simulink model "eBooster_48v_Gen2_r2009a"  (Simulink 7.6)
settings: Solver=FixedStepDiscrete  StartTime=0.0  StopTime=0.2  FixedStep=T_sim  RelTol=1e-3
InitFcn:
  | init_simulation
values from neighbouring files (symbols this model uses):
  C_Load = 0    [init_MIL.m]    (also in init_simulation.m)
  curr_adc_gain = 0.6247    [init_MIL.m]    (also in init_simulation.m)
  en_avr = 0    [init_MIL.m]    (also in init_simulation.m)
  FOC_CURR_GAIN_SCU10 = 640    [init_MIL.m]    (also in init_simulation.m)
  FOC_CURR_NULLIFICATION = 511    [init_MIL.m]    (also in init_simulation.m)
  I_max = 106    [init_MIL.m]    (also in init_simulation.m = 100; plot_current_limits.m = 160)
  Id_ref_min = -1*160*0.8    (= -128)    [init_MIL.m]    (also in init_simulation.m)
  J_motor = (3.2220 + 11.438)*1e-6    (= 1.466e-05)    [init_MIL.m]    (also in init_simulation.m)
  Kpi = 0.3    [init_MIL.m]    (also in init_simulation.m)
  Kpi_n = 0.0015    [init_MIL.m]    (also in init_simulation.m)
  load_motor_spd_ramp = (load_motor_target_spd - load_motor_start_spd)/spd_ramp_time    (= 62831.8530718)    [init_MIL.m]    (also in init_simulation.m)
  load_motor_start_spd = 40000*2*pi/60    (= 4188.79020479)    [init_MIL.m]    (also in init_simulation.m)
  load_motor_target_spd = 70000*2*pi/60    (= 7330.38285838)    [init_MIL.m]    (also in init_simulation.m)
  Ls = 17.05e-6/3    (= 5.68333333333e-06)    [init_MIL.m]    (also in init_simulation.m; plot_current_limits.m)
  N_avr = 1    [init_MIL.m]    (also in init_simulation.m)
  Nset_const = 50000    [init_MIL.m]    (also in init_simulation.m)
  ONEDIVSQRT3_SCU16 = 37837    [init_MIL.m]    (also in init_simulation.m)
  Pp = 1    [init_MIL.m]    (also in init_simulation.m; plot_current_limits.m)
  psi_p = 5.3e-3/sqrt(3)*0.95    [init_MIL.m]    (also in init_simulation.m)
  Rs = 10e-3*(1+0.0039*(120-20))/3    (= 0.00463333333333)    [init_MIL.m]    (also in init_simulation.m; plot_current_limits.m)
  Sel_Bench_Mode = 1    [init_MIL.m]    (also in init_simulation.m)
  Sel_Bench_Spd = 0    [init_MIL.m]    (also in init_simulation.m)
  Sel_id_ref = 2    [init_MIL.m]    (also in init_simulation.m)
  Sel_Load = 1    [init_MIL.m]    (also in init_simulation.m)
  sel_udq = 0    [init_simulation.m]
  Set_Speed_rpm = 50000    [init_MIL.m]    (also in init_simulation.m)
  T_ctrl = T_pwm    (= 3.57002606119e-05)    [init_MIL.m]    (also in init_simulation.m)
  T_LUT_T = [0.1864, 0.1969, 0.2092, 0.2230, 0.2381, 0.2541, 0.2709, 0.2880, 0.3054, 0.3226, 0.3395, 0.3557, 0.3710, 0.3851, 0.3978, 0.4088, 0.4178 ... (first row only)    [init_MIL.m]    (also in init_simulation.m)
  T_sim = T_pwm/100    (= 3.57002606119e-07)    [init_MIL.m]    (also in init_simulation.m)
  Tni = Ts    (= 0.00122661870504)    [init_MIL.m]    (also in init_simulation.m)
  Tni_n = Ts*1.5    (= 0.00183992805755)    [init_MIL.m]    (also in init_simulation.m)
  V_dc = 36    [init_MIL.m]    (also in init_simulation.m)
libraries: simulink x27
(part 2 of 2)

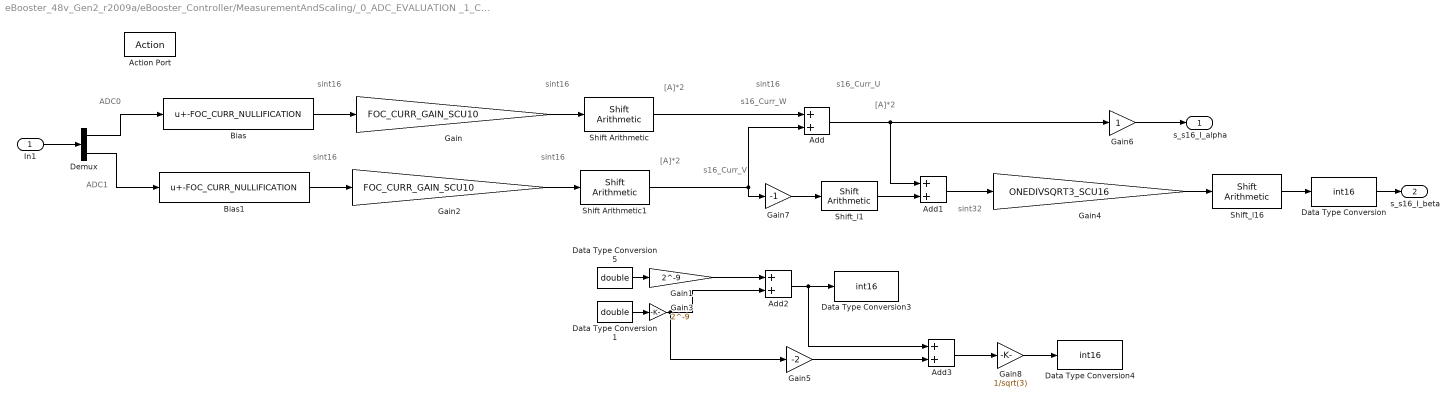
== system eBooster_48v_Gen2_r2009a/eBooster_Controller/MeasurementAndScaling/_0_ADC_EVALUATION _1_CLARKE_TRANSFORMATION1/sector_1_6 ==
  note: ADC1
  note: sint32
  note: s16_Curr_V
  note: s16_Curr_W
  note: [A]*2
  note: s16_Curr_U
  note: sint16
  note: sint16
  note: [A]*2
  note: sint16
  note: sint16
  note: sint16
  note: [A]*2
  note: ADC0
  In1 : Inport
  Action Port : ActionPort  PropagateVarSize=During execution
  Add : Sum  OutDataTypeStr=int16
  Add1 : Sum  AccumDataTypeStr=int32  OutDataTypeStr=int32
  Add2 : Sum  OutDataTypeStr=double
  Add3 : Sum  OutDataTypeStr=double
  Bias : Bias  Bias=-FOC_CURR_NULLIFICATION
  Bias1 : Bias  Bias=-FOC_CURR_NULLIFICATION
  Data Type Conversion : DataTypeConversion  OutDataTypeStr=int16
  Data Type Conversion1 : DataTypeConversion  OutDataTypeStr=double
  Data Type Conversion3 : DataTypeConversion  OutDataTypeStr=int16
  Data Type Conversion4 : DataTypeConversion  OutDataTypeStr=int16
  Data Type Conversion5 : DataTypeConversion  OutDataTypeStr=double
  Demux : Demux  Outputs=2
  Gain : Gain  Gain=FOC_CURR_GAIN_SCU10  ParamDataTypeStr=uint16  OutDataTypeStr=int32
  Gain1 : Gain  Gain=2^-9  OutDataTypeStr=double
  Gain2 : Gain  Gain=FOC_CURR_GAIN_SCU10  ParamDataTypeStr=uint16  OutDataTypeStr=int32
  Gain3 : Gain  Gain=2^-9  OutDataTypeStr=double
  Gain4 : Gain  Gain=ONEDIVSQRT3_SCU16  OutDataTypeStr=int32
  Gain5 : Gain  Gain=-2  OutDataTypeStr=double
  Gain6 : Gain  OutDataTypeStr=int16
  Gain7 : Gain  Gain=-1  ParamDataTypeStr=int32  OutDataTypeStr=int16
  Gain8 : Gain  Gain=1/sqrt(3)  OutDataTypeStr=double
  Shift Arithmetic : simulink/Logic and Bit Operations/Shift Arithmetic  SystemSampleTime=-1  nBitShiftRight=9  nBinPtShiftRight=0
  Shift Arithmetic1 : simulink/Logic and Bit Operations/Shift Arithmetic  SystemSampleTime=-1  nBitShiftRight=9  nBinPtShiftRight=0
  Shift_l1 : simulink/Logic and Bit Operations/Shift Arithmetic  SystemSampleTime=-1  nBitShiftRight=-1  nBinPtShiftRight=0
  Shift_l16 : simulink/Logic and Bit Operations/Shift Arithmetic  SystemSampleTime=-1  nBitShiftRight=16  nBinPtShiftRight=0
  s_s16_I_alpha : Outport
  s_s16_I_beta : Outport  Port=2
  wires:
  Gain7/1 -> Shift_l1/1
  Shift_l16/1 -> Data Type Conversion/1
  Gain4/1 -> Shift_l16/1
  Add1/1 -> Gain4/1
  Shift_l1/1 -> Add1/2
  Add/1 -> Gain6/1, Add1/1
  Demux/2 -> Bias1/1
  Shift Arithmetic1/1 -> Gain7/1, Add/2
  Gain2/1 -> Shift Arithmetic1/1
  Bias1/1 -> Gain2/1
  Shift Arithmetic/1 -> Add/1
  Gain/1 -> Shift Arithmetic/1
  Bias/1 -> Gain/1
  Demux/1 -> Bias/1
  In1/1 -> Demux/1
  Add2/1 -> Data Type Conversion3/1, Add3/1
  Gain5/1 -> Add3/2
  Add3/1 -> Gain8/1
  Gain8/1 -> Data Type Conversion4/1
  Data Type Conversion5/1 -> Gain1/1
  Data Type Conversion1/1 -> Gain3/1
  Gain1/1 -> Add2/1
  Gain3/1 -> Add2/2, Gain5/1
  Gain6/1 -> s_s16_I_alpha/1
  Data Type Conversion/1 -> s_s16_I_beta/1

== system eBooster_48v_Gen2_r2009a/eBooster_Controller/MeasurementAndScaling/_0_ADC_EVALUATION _1_CLARKE_TRANSFORMATION1/sector_2_3 ==
  note: [A]*2
  note: s16_Curr_W
  note: s16_Curr_U
  note: s16_Curr_V
  note: sint32
  note: ADC0
  note: [A]*2
  note: sint16
  note: sint16
  note: sint16
  note: [A]*2
  note: sint16
  note: sint16
  In1 : Inport
  Action Port : ActionPort  PropagateVarSize=During execution
  Add : Sum  OutDataTypeStr=int16
  Add2 : Sum  AccumDataTypeStr=int32  OutDataTypeStr=int32
  Bias : Bias  Bias=-FOC_CURR_NULLIFICATION
  Bias1 : Bias  Bias=-FOC_CURR_NULLIFICATION
  Data Type Conversion : DataTypeConversion  OutDataTypeStr=int16
  Demux : Demux  Outputs=2
  Gain : Gain  Gain=FOC_CURR_GAIN_SCU10  OutDataTypeStr=int32
  Gain1 : Gain  Gain=-1  ParamDataTypeStr=int32  OutDataTypeStr=int16
  Gain2 : Gain  Gain=FOC_CURR_GAIN_SCU10  OutDataTypeStr=int32
  Gain3 : Gain  Gain=-1  ParamDataTypeStr=int32  OutDataTypeStr=int16
  Gain4 : Gain  Gain=ONEDIVSQRT3_SCU16  OutDataTypeStr=int32
  Gain5 : Gain  Gain=-1  ParamDataTypeStr=int32
  Gain6 : Gain  OutDataTypeStr=int16
  Shift Arithmetic : simulink/Logic and Bit Operations/Shift Arithmetic  SystemSampleTime=-1  nBitShiftRight=9  nBinPtShiftRight=0
  Shift Arithmetic1 : simulink/Logic and Bit Operations/Shift Arithmetic  SystemSampleTime=-1  nBitShiftRight=9  nBinPtShiftRight=0
  Shift_l1 : simulink/Logic and Bit Operations/Shift Arithmetic  SystemSampleTime=-1  nBitShiftRight=-1  nBinPtShiftRight=0
  Shift_l16 : simulink/Logic and Bit Operations/Shift Arithmetic  SystemSampleTime=-1  nBitShiftRight=16  nBinPtShiftRight=0
  s_s16_I_alpha : Outport
  s_s16_I_beta : Outport  Port=2
  wires:
  Gain6/1 -> s_s16_I_alpha/1
  Gain5/1 -> Shift_l1/1
  Data Type Conversion/1 -> s_s16_I_beta/1
  Add/1 -> Gain5/1
  Shift_l16/1 -> Data Type Conversion/1
  Gain4/1 -> Shift_l16/1
  Add2/1 -> Gain4/1
  Shift_l1/1 -> Add2/2
  In1/1 -> Demux/1
  Bias/1 -> Gain/1
  Gain/1 -> Shift Arithmetic/1
  Shift Arithmetic/1 -> Gain1/1
  Gain1/1 -> Gain6/1, Add2/1, Add/1
  Bias1/1 -> Gain2/1
  Gain2/1 -> Shift Arithmetic1/1
  Shift Arithmetic1/1 -> Gain3/1
  Gain3/1 -> Add/2
  Demux/1 -> Bias1/1
  Demux/2 -> Bias/1

== system eBooster_48v_Gen2_r2009a/eBooster_Controller/MeasurementAndScaling/_0_ADC_EVALUATION _1_CLARKE_TRANSFORMATION1/sector_4_5 ==
  note: sint16
  note: s16_Curr_U
  note: s16_Curr_V
  note: sint32
  note: sint16
  note: sint16
  note: [A]*2
  note: sint16
  note: sint16
  note: [A]*2
  note: ADC0
  In1 : Inport
  Action Port : ActionPort  PropagateVarSize=During execution
  Add2 : Sum  AccumDataTypeStr=int32  OutDataTypeStr=int32
  Bias : Bias  Bias=-FOC_CURR_NULLIFICATION
  Bias1 : Bias  Bias=-FOC_CURR_NULLIFICATION
  Data Type Conversion : DataTypeConversion  OutDataTypeStr=int16
  Demux : Demux  Outputs=2
  Gain : Gain  Gain=FOC_CURR_GAIN_SCU10  OutDataTypeStr=int32
  Gain1 : Gain  Gain=-1  ParamDataTypeStr=int32  OutDataTypeStr=int16
  Gain2 : Gain  Gain=FOC_CURR_GAIN_SCU10  OutDataTypeStr=int32
  Gain3 : Gain  Gain=-1  ParamDataTypeStr=int32  OutDataTypeStr=int16
  Gain4 : Gain  Gain=ONEDIVSQRT3_SCU16  OutDataTypeStr=int32
  Gain6 : Gain  OutDataTypeStr=int16
  Shift Arithmetic : simulink/Logic and Bit Operations/Shift Arithmetic  SystemSampleTime=-1  nBitShiftRight=9  nBinPtShiftRight=0
  Shift Arithmetic1 : simulink/Logic and Bit Operations/Shift Arithmetic  SystemSampleTime=-1  nBitShiftRight=9  nBinPtShiftRight=0
  Shift_l1 : simulink/Logic and Bit Operations/Shift Arithmetic  SystemSampleTime=-1  nBitShiftRight=-1  nBinPtShiftRight=0
  Shift_l16 : simulink/Logic and Bit Operations/Shift Arithmetic  SystemSampleTime=-1  nBitShiftRight=16  nBinPtShiftRight=0
  s_s16_I_alpha : Outport
  s_s16_I_beta : Outport  Port=2
  wires:
  Gain6/1 -> s_s16_I_alpha/1
  Data Type Conversion/1 -> s_s16_I_beta/1
  Shift_l16/1 -> Data Type Conversion/1
  Gain4/1 -> Shift_l16/1
  Add2/1 -> Gain4/1
  Shift_l1/1 -> Add2/2
  Gain3/1 -> Shift_l1/1
  Demux/2 -> Bias1/1
  Shift Arithmetic1/1 -> Gain3/1
  Gain2/1 -> Shift Arithmetic1/1
  Bias1/1 -> Gain2/1
  Gain1/1 -> Gain6/1, Add2/1
  Shift Arithmetic/1 -> Gain1/1
  Gain/1 -> Shift Arithmetic/1
  Bias/1 -> Gain/1
  Demux/1 -> Bias/1
  In1/1 -> Demux/1

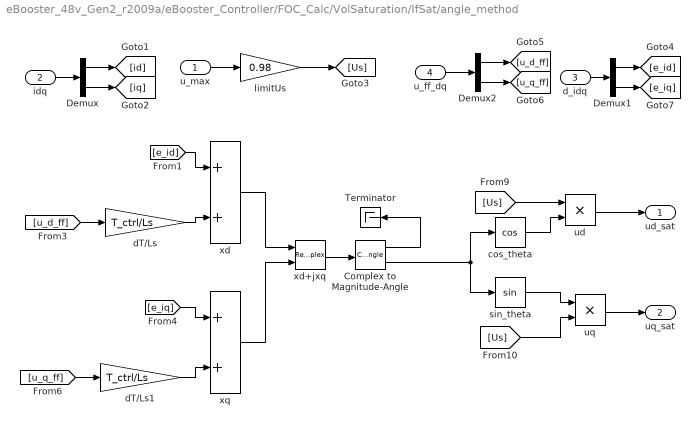
== system eBooster_48v_Gen2_r2009a/eBooster_Controller/FOC_Calc/VolSaturation/IfSat/angle_method ==
  u_max : Inport
  idq : Inport  Port=2
  d_idq : Inport  Port=3
  u_ff_dq : Inport  Port=4
  Complex to Magnitude-Angle : ComplexToMagnitudeAngle
  Demux : Demux  Outputs=2
  Demux1 : Demux  Outputs=2
  Demux2 : Demux  Outputs=2
  Terminator : Terminator
  cos_theta : Trigonometry  Operator=cos
  dT/Ls : Gain  Gain=T_ctrl/Ls
  dT/Ls1 : Gain  Gain=T_ctrl/Ls
  limitUs : Gain  Gain=0.98
  sin_theta : Trigonometry
  ud : Product  RndMeth=Zero
  uq : Product  RndMeth=Zero
  xd : Sum
  xd+jxq : RealImagToComplex
  xq : Sum
  ud_sat : Outport
  uq_sat : Outport  Port=2
  wires:
  idq/1 -> Demux/1
  d_idq/1 -> Demux1/1
  Demux/1 -> [id]
  Demux/2 -> [iq]
  u_max/1 -> limitUs/1
  Complex to Magnitude-Angle/2 -> cos_theta/1, sin_theta/1
  [Us] -> ud/1
  cos_theta/1 -> ud/2
  sin_theta/1 -> uq/1
  [Us] -> uq/2
  Demux2/1 -> [u_d_ff]
  Demux2/2 -> [u_q_ff]
  u_ff_dq/1 -> Demux2/1
  Demux1/1 -> [e_id]
  Demux1/2 -> [e_iq]
  [e_id] -> xd/1
  dT/Ls/1 -> xd/2
  [u_d_ff] -> dT/Ls/1
  [e_iq] -> xq/1
  dT/Ls1/1 -> xq/2
  [u_q_ff] -> dT/Ls1/1
  xd/1 -> xd+jxq/1
  xq/1 -> xd+jxq/2
  xd+jxq/1 -> Complex to Magnitude-Angle/1
  Complex to Magnitude-Angle/1 -> Terminator/1
  ud/1 -> ud_sat/1
  uq/1 -> uq_sat/1
  limitUs/1 -> [Us]

== system eBooster_48v_Gen2_r2009a/eBooster_Controller/FOC_Calc/VolSaturation/IfSat/d_priority ==
  udq : Inport
  u_max : Inport  Port=2
  Abs : Abs
  Demux : Demux  Outputs=2
  Gain : Gain  Gain=-1
  Product : Product  RndMeth=Zero
  Product1 : Product  RndMeth=Zero
  Product2 : Product  RndMeth=Zero
  Saturation Dynamic : simulink/Discontinuities/Saturation Dynamic  SystemSampleTime=-1  OutMin=[]  OutMax=[]  OutDataTypeStr=Inherit: Same as second input  OutDataType=fixdt(1, 16)  OutScaling=2^-10  DoSatur=off
  Sign : Signum
  Sqrt : Math  Operator=sqrt  SaturateOnIntegerOverflow=on
  Subtract : Sum  Inputs=-+
  ud_sat : Outport
  uq_sat : Outport  Port=2
  wires:
  u_max/1 -> Product1/1, Product1/2, Saturation Dynamic/1, Gain/1
  Product/1 -> Subtract/1
  Product1/1 -> Subtract/2
  Subtract/1 -> Abs/1
  Saturation Dynamic/1 -> Product/1, Product/2, ud_sat/1
  Gain/1 -> Saturation Dynamic/3
  Sqrt/1 -> Product2/1
  udq/1 -> Demux/1
  Demux/1 -> Saturation Dynamic/2
  Demux/2 -> Sign/1
  Sign/1 -> Product2/2
  Product2/1 -> uq_sat/1
  Abs/1 -> Sqrt/1
